simulink model "pp"  (R2013b)
settings: Solver=ode3  StartTime=0.0  StopTime=100  FixedStep=0.01  RelTol=1e-3
libraries: simulink x1
settings Model: Creator=Bara Emran  LastModifiedBy=Bara Emran

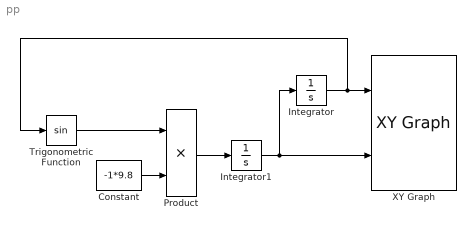
== system pp ==
  Constant : Constant  Value=-1*9.8
  Integrator : Integrator  InitialCondition=pi-1
  Integrator1 : Integrator  InitialCondition=0.5
  Product : Product
  Trigonometric Function : Trigonometry
  XY Graph : simulink/Sinks/XY Graph  xmin=-15  xmax=15  ymin=-10  ymax=10  st=-1
  wires:
  Integrator1/1 -> XY Graph/2, Integrator/1
  Constant/1 -> Product/2
  Trigonometric Function/1 -> Product/1
  Integrator/1 -> Trigonometric Function/1, XY Graph/1
  Product/1 -> Integrator1/1
